simulink model "sampleModel339"  (R2021b)
settings: Solver=VariableStepAuto  StartTime=0.0  StopTime=10.0  RelTol=1e-3
undefined symbols (not defined in the file or in its folder): DiscIntNeverNeededParam
libraries: simulink x5
settings Model: Creator=user  LastModifiedBy=user

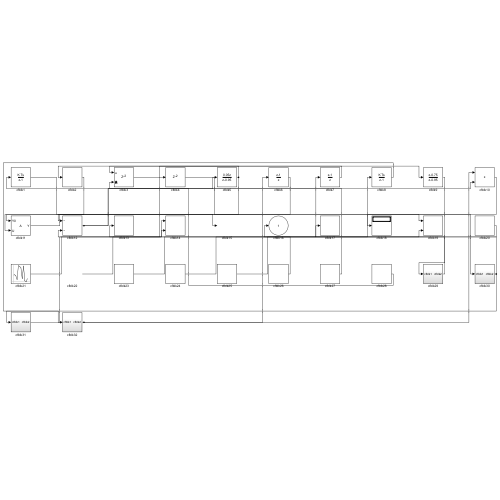
[thumbnail: Simulink's stored preview of the top-level diagram]
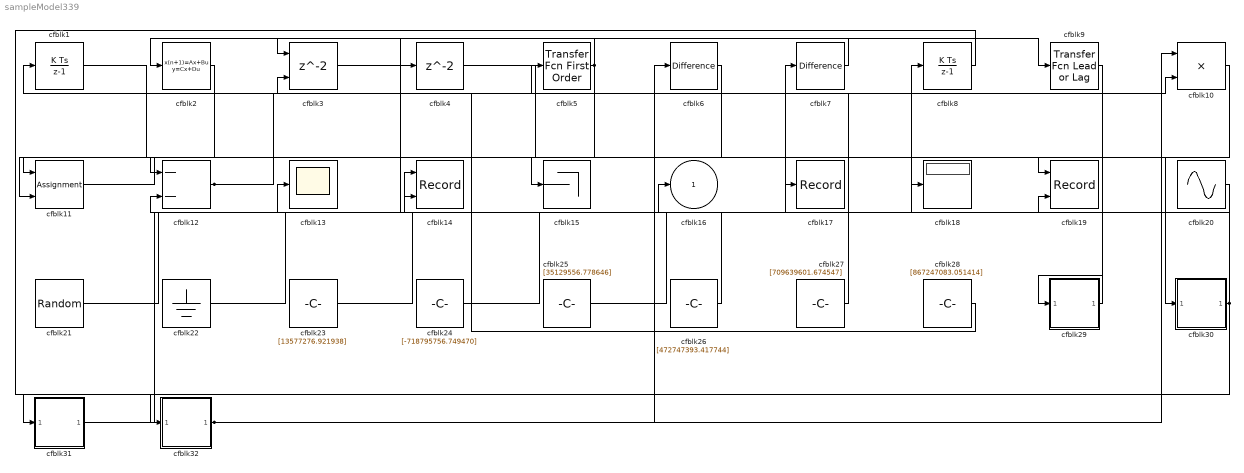
== system sampleModel339 ==
  cfblk1 : DiscreteIntegrator  ICPrevOutput=DiscIntNeverNeededParam  ICPrevScaledInput=DiscIntNeverNeededParam
  cfblk10 : Product  Inputs=**
  cfblk11 : Assignment  DiagnosticForDimensions=Warning  IndexOptions=Index vector (dialog)  Indices=1  OutputSizes=1
  cfblk12 : Sum  Inputs=--
  cfblk13 : Scope
  cfblk14 : Record  FileSettingsInternal="{\"entries\":[{\"content\":{\"excelSettings\":{\"content\":{},\"type\":\"Streamout.ExcelSettings\"}},\"type\":\"Streamout.FileSettingStorage\",\"uuid\":\"70ba667a-bbb0-4f1f-9711-881f65f82685\"}],\"packageUris\":[\"http://schema.mathworks.com/mf0/streamout_blocks/R2020a\"],\"version\":\"1.0\"}"  Layout=[1 1]  SignalsInternal="{\"entries\":[{\"content\":{\"signals\":[{\"content\":{\"blockPath\":[\"sampleModel339/cfblk14\"],\"channel\":[],\"dimensions\":[1],\"domain\":\"sampleModel339/cfblk14\",\"lineColor\":\"#a2142f\",\"plots\":[1],\"port\":1,\"sid\":[\"\"],\"signalID\":14289,\"signalName\":\"cfblk31\"},\"type\":\"RecordBlkView.Signal\",\"uuid\":\"780fe4fa-e180-4cf4-aaa4-dc4569e8b29f\"},{\"content\":{\"blockPath\":[\"sampleModel339/cfblk14\"],\"channel\":[],\"dimensions\":[1],\"domain\":\"sampleModel339/cfblk14\",\"lineColor\":\"#139fff\",\"plots\":[1],\"port\":2,\"sid\":[\"\"],\"signalID\":14293,\"signalName\":\"cfblk21\"},\"type\":\"RecordBlkView.Signal\",\"uuid\":\"335cd3bc-e225-4aff-bc5a-e98ec1313b65\"}]},\"type\":\"RecordBlkView.InputSignals\",\"uuid\":\"db6856a2-41bb-4a85-a1f6-148ec1af43ec\"}],\"packageUris\":[\"http://schema.mathworks.com/mf0/streamout_blocks/R2020a\"],\"version\":\"1.0\"}"  VisualizationBindings="{\"xyplotplugin\":{\"info\":[{\"series\":[{\"bindingParametersList\":[{\"parameter\":\"X-Axis\",\"signalID\":14289,\"signalName\":\"cfblk31\"},{\"parameter\":\"Y-Axis\",\"signalID\":14293,\"signalName\":\"cfblk21\"}],\"seriesID\":63424}],\"subplotID\":1}]}}"  CompatibilityTag=XY
  cfblk15 : Terminator
  cfblk17 : Record  FileSettingsInternal="{\"entries\":[{\"content\":{\"excelSettings\":{\"content\":{},\"type\":\"Streamout.ExcelSettings\"}},\"type\":\"Streamout.FileSettingStorage\",\"uuid\":\"f29af9df-93c7-46ee-88f2-aed450e863f6\"}],\"packageUris\":[\"http://schema.mathworks.com/mf0/streamout_blocks/R2020a\"],\"version\":\"1.0\"}"  SignalsInternal="{\"entries\":[{\"content\":{\"signals\":[{\"content\":{\"blockPath\":[\"sampleModel339/cfblk17\"],\"channel\":[],\"dimensions\":[1],\"domain\":\"sampleModel339/cfblk17\",\"lineColor\":\"#edb120\",\"plots\":[1],\"port\":1,\"sid\":[\"\"],\"signalID\":14297,\"signalName\":\"cfblk30\"},\"type\":\"RecordBlkView.Signal\",\"uuid\":\"7d3e7fc6-6dd4-4698-b0e0-03b653032e45\"}]},\"type\":\"RecordBlkView.InputSignals\",\"uuid\":\"0b41b631-07f1-4357-a455-e4717be9e647\"}],\"packageUris\":[\"http://schema.mathworks.com/mf0/streamout_blocks/R2020a\"],\"version\":\"1.0\"}"  VisualizationBindings="{\"sparklinesplugin\":{\"info\":[{\"bindingParametersList\":[],\"subplotID\":1}]}}"
  cfblk18 : Display
  cfblk19 : Record  FileSettingsInternal="{\"entries\":[{\"content\":{\"excelSettings\":{\"content\":{},\"type\":\"Streamout.ExcelSettings\"}},\"type\":\"Streamout.FileSettingStorage\",\"uuid\":\"24023120-a528-49a7-a403-18bd6bee5134\"}],\"packageUris\":[\"http://schema.mathworks.com/mf0/streamout_blocks/R2020a\"],\"version\":\"1.0\"}"  Layout=[1 1]  SignalsInternal="{\"entries\":[{\"content\":{\"signals\":[{\"content\":{\"blockPath\":[\"sampleModel339/cfblk19\"],\"channel\":[],\"dimensions\":[1],\"domain\":\"sampleModel339/cfblk19\",\"lineColor\":\"#a2142f\",\"plots\":[1],\"port\":1,\"sid\":[\"\"],\"signalID\":14281,\"signalName\":\"cfblk11\"},\"type\":\"RecordBlkView.Signal\",\"uuid\":\"e47dcd13-cce1-47c4-b0b2-d82808c5e28b\"},{\"content\":{\"blockPath\":[\"sampleModel339/cfblk19\"],\"channel\":[],\"dimensions\":[1],\"domain\":\"sampleModel339/cfblk19\",\"lineColor\":\"#139fff\",\"plots\":[1],\"port\":2,\"sid\":[\"\"],\"signalID\":14285,\"signalName\":\"cfblk23\"},\"type\":\"RecordBlkView.Signal\",\"uuid\":\"cdbc505c-56be-4969-be2d-752a4e318810\"}]},\"type\":\"RecordBlkView.InputSignals\",\"uuid\":\"69bbe3dd-b93b-4d7f-9466-3fa7cd078233\"}],\"packageUris\":[\"http://schema.mathworks.com/mf0/streamout_blocks/R2020a\"],\"version\":\"1.0\"}"  VisualizationBindings="{\"xyplotplugin\":{\"info\":[{\"series\":[{\"bindingParametersList\":[{\"parameter\":\"X-Axis\",\"signalID\":14281,\"signalName\":\"cfblk11\"},{\"parameter\":\"Y-Axis\",\"signalID\":14285,\"signalName\":\"cfblk23\"}],\"seriesID\":55003}],\"subplotID\":1}]}}"  CompatibilityTag=XY
  cfblk2 : DiscreteStateSpace
  cfblk20 : Sin  Amplitude=[-171637283.497394]  Bias=[374292158.541033]  SampleTime=0
  cfblk21 : RandomNumber  Mean=[72096.763381]  Variance=[14588.051510]  Seed=[504940882.000000]  SampleTime=0.1
  cfblk22 : Ground
  cfblk23 : Constant  Value=[13577276.921938]  SampleTime=1
  cfblk24 : Constant  Value=[-718795756.749470]  SampleTime=1
  cfblk25 : Constant  Value=[35129556.778646]  SampleTime=1
  cfblk26 : Constant  Value=[472747393.417744]  SampleTime=1
  cfblk27 : Constant  Value=[709639601.674547]  SampleTime=1
  cfblk28 : Constant  Value=[867247083.051414]  SampleTime=1
  cfblk29 : Subsystem
  cfblk3 : Delay  ShowEnablePort=on  SampleTime=1
      settings: InputPortMap=u0,e6
  cfblk30 : Subsystem
  cfblk31 : Subsystem
  cfblk32 : Subsystem
  cfblk4 : Delay  SampleTime=1
  cfblk5 : simulink/Discrete/Transfer Fcn First Order  PoleZ=0.95  ICPrevOutput=0.0  DoSatur=off
  cfblk6 : simulink/Discrete/Difference  ICPrevInput=0.0  OutMin=[]  OutMax=[]  OutDataTypeStr=Inherit: Inherit via back propagation  OutDataType=fixdt(1, 16)  OutScaling=2^-10  DoSatur=off
  cfblk7 : simulink/Discrete/Difference  ICPrevInput=0.0  OutMin=[]  OutMax=[]  OutDataTypeStr=Inherit: Inherit via back propagation  OutDataType=fixdt(1, 16)  OutScaling=2^-10  DoSatur=off
  cfblk8 : DiscreteIntegrator  ICPrevOutput=DiscIntNeverNeededParam  ICPrevScaledInput=DiscIntNeverNeededParam
  cfblk9 : simulink/Discrete/Transfer Fcn Lead or Lag  PoleZ=0.95  ZeroZ=0.75  ICPrevOutput=0.0  ICPrevInput=0.0  DoSatur=off
      settings: SourceProductBaseCode=SL
  cfblk16 : Outport
  wires:
  cfblk26/1 -> cfblk16/1
  cfblk31/1(cfblk2) -> cfblk14/1
  cfblk4/1 -> cfblk30/1(cfblk1)
  cfblk28/1 -> cfblk1/1
  cfblk9/1 -> cfblk29/1(cfblk1)
  cfblk11/1 -> cfblk19/1
  cfblk29/1(cfblk2) -> cfblk13/1
  cfblk7/1 -> cfblk2/1
  cfblk12/1 -> cfblk5/1, cfblk10/2
  cfblk5/1 -> cfblk3/1, cfblk11/2
  cfblk8/1 -> cfblk32/1(cfblk1)
  cfblk23/1 -> cfblk19/2
  cfblk25/1 -> cfblk8/1
  cfblk22/1 -> cfblk4/1
  cfblk1/1 -> cfblk15/1
  cfblk21/1 -> cfblk14/2
  cfblk24/1 -> cfblk7/1
  cfblk2/1 -> cfblk12/1
  cfblk27/1 -> cfblk3/2
  cfblk32/1(cfblk2) -> cfblk6/1, cfblk10/1
  cfblk10/1 -> cfblk18/1
  cfblk20/1 -> cfblk12/2
  cfblk30/1(cfblk2) -> cfblk17/1, cfblk31/1(cfblk1)
  cfblk6/1 -> cfblk11/1
  cfblk3/1 -> cfblk9/1

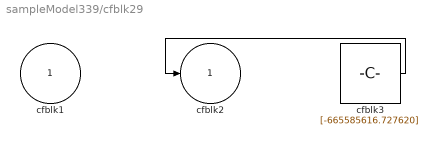
== system sampleModel339/cfblk29 ==
  cfblk1 : Inport
  cfblk3 : Constant  Value=[-665585616.727620]  SampleTime=1
  cfblk2 : Outport
  wires:
  cfblk3/1 -> cfblk2/1

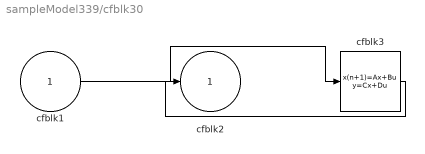
== system sampleModel339/cfblk30 ==
  cfblk1 : Inport
  cfblk3 : DiscreteStateSpace
  cfblk2 : Outport
  wires:
  cfblk1/1 -> cfblk3/1
  cfblk3/1 -> cfblk2/1

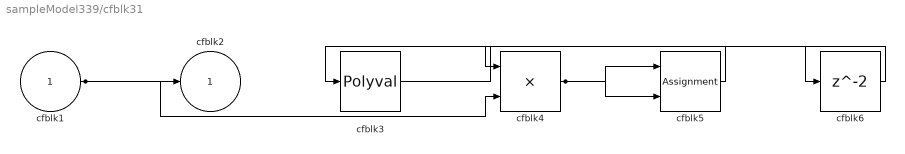
== system sampleModel339/cfblk31 ==
  cfblk1 : Inport
  cfblk3 : Polyval  Coefs=[ +2.081618890e-019, -1.441693666e-014, +4.719686976e-010, -8.536869453e-006, +1.621573104e-001, -8.087801117e+001 ]
  cfblk4 : Product  Inputs=**
  cfblk5 : Assignment  DiagnosticForDimensions=Warning  IndexOptions=Index vector (dialog)  Indices=1  OutputSizes=1
  cfblk6 : Delay  SampleTime=1
  cfblk2 : Outport
  wires:
  cfblk5/1 -> cfblk3/1
  cfblk1/1 -> cfblk2/1, cfblk4/2
  cfblk4/1 -> cfblk5/1, cfblk5/2
  cfblk3/1 -> cfblk6/1
  cfblk6/1 -> cfblk4/1

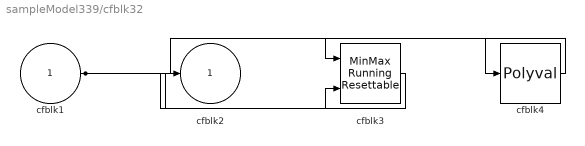
== system sampleModel339/cfblk32 ==
  cfblk1 : Inport
  cfblk3 : simulink/Math Operations/MinMax Running Resettable  Function=min  vinit=0.0
  cfblk4 : Polyval  Coefs=[ +2.081618890e-019, -1.441693666e-014, +4.719686976e-010, -8.536869453e-006, +1.621573104e-001, -8.087801117e+001 ]
  cfblk2 : Outport
  wires:
  cfblk1/1 -> cfblk4/1, cfblk3/2
  cfblk3/1 -> cfblk2/1
  cfblk4/1 -> cfblk3/1
